simulink model "CAR_CONTROL_SYSTEM"  (R2024b)
settings: Solver=FixedStepAuto  StartTime=0.0  StopTime=inf  FixedStep=1e-3  RelTol=1e-3  EnableMultiTasking=on
model workspace (MAT data in the model file):
  SL_ROS_VariableLengthArrays_MaxSizes : object (value not decoded)
undefined symbols (not defined in the file or in its folder): angular, CIRCUIT, CLTF_DAMP, CLTF_FREQ, CLTF_GAIN, CONTROL, CONTROL_INI, DiscIntNeverNeededParam, dspblkCoreblockFVToolHelper, gcbh, INPUT, linear, MCP3201, MD25, MODEL, MODEL_INI, mpcstate, MPU60X0, MPU9250, MSG, NAV_MPC_CONTROL, OUTPUT, SAMPLING_TIME, SYSID_INPUT, VL6180X
libraries: raspberrypiCommlib x153, simulink x85, raspberrypiNetworklib x8, embedlinuxBasiclib x6, ctrlSharedLib x2, ros2lib x2, mpclib x1, vrlib x1, sldrtlib x1
(part 8 of 16)

== system CAR_CONTROL_SYSTEM/HARDWARE/SENSORS/WALL RANGE SENSOR/VL6180X_I2C_FRONT/VL6180X INITIALIZATION/MEASUREMENT CONFIGURATION/START READ RANGE CONTINUOUS ==
  Enable : EnablePort
  Constant2 : Constant  Value=hex2dec('03')  OutDataTypeStr=uint8  SampleTime=SAMPLING_TIME
  I2C WRITE: SYSRANGE_START : Subsystem  mask{SLAVE_ADDRESS=VL6180X.ADDRESS, REGISTER_ADDRESS=VL6180X.SYSRANGE_START}
      mask prompts: SLAVE_ADDRESS "SLAVE ADDRESS"; REGISTER_ADDRESS "REGISTER ADDRESS"
      mask init:
      | REGISTER_ADDRESS_MSB = uint8(floor(REGISTER_ADDRESS/(2^8)));
      | REGISTER_ADDRESS_LSB = uint8(rem(REGISTER_ADDRESS,2^8));
  wires:
  Constant2/1 -> I2C WRITE: SYSRANGE_START/1(DATA)

== system CAR_CONTROL_SYSTEM/HARDWARE/SENSORS/WALL RANGE SENSOR/VL6180X_I2C_FRONT/VL6180X INITIALIZATION/MEASUREMENT CONFIGURATION/START READ RANGE SINGLE ==
  Enable : EnablePort
  Constant1 : Constant  Value=hex2dec('01')  OutDataTypeStr=uint8  SampleTime=SAMPLING_TIME
  I2C WRITE: SYSRANGE_START : Subsystem  mask{SLAVE_ADDRESS=VL6180X.ADDRESS, REGISTER_ADDRESS=VL6180X.SYSRANGE_START}
      mask prompts: SLAVE_ADDRESS "SLAVE ADDRESS"; REGISTER_ADDRESS "REGISTER ADDRESS"
      mask init:
      | REGISTER_ADDRESS_MSB = uint8(floor(REGISTER_ADDRESS/(2^8)));
      | REGISTER_ADDRESS_LSB = uint8(rem(REGISTER_ADDRESS,2^8));
  wires:
  Constant1/1 -> I2C WRITE: SYSRANGE_START/1(DATA)

== system CAR_CONTROL_SYSTEM/HARDWARE/SENSORS/WALL RANGE SENSOR/VL6180X_I2C_FRONT/VL6180X INITIALIZATION/OTHER SPECIFIC SETTINGS (OPTIONAL)/I2C WRITE: INTERLEAVED_MODE_ENABLE ==
  DATA : Inport
  Constant : Constant  Value=REGISTER_ADDRESS_MSB  OutDataTypeStr=uint8  SampleTime=SAMPLING_TIME
  Constant1 : Constant  Value=REGISTER_ADDRESS_LSB  OutDataTypeStr=uint8  SampleTime=SAMPLING_TIME
  Mux : Mux  Inputs=3
  REGISTER ADDRESS : raspberrypiCommlib/I2C Controller Write  Priority=10  BoardProperty=Pi 3 Model B+  I2CModule=1  Mode=Master  SlaveAddress=SLAVE_ADDRESS  SlaveByteOrder=BigEndian  Direction=Transmitter  RegisterAddressMode=off  RegisterAddress=hex2dec('207')  SlaveDataType=uint8  DataLength=1  NoAck=off  RepeatedStart=off  OutputStatus=off
  wires:
  Mux/1 -> REGISTER ADDRESS/1
  Constant/1 -> Mux/1
  DATA/1 -> Mux/3
  Constant1/1 -> Mux/2

== system CAR_CONTROL_SYSTEM/HARDWARE/SENSORS/WALL RANGE SENSOR/VL6180X_I2C_FRONT/VL6180X INITIALIZATION/OTHER SPECIFIC SETTINGS (OPTIONAL)/I2C WRITE: SYSRANGE_MAX_CONVERGENCE_TIME ==
  DATA : Inport
  Constant : Constant  Value=REGISTER_ADDRESS_MSB  OutDataTypeStr=uint8  SampleTime=SAMPLING_TIME
  Constant1 : Constant  Value=REGISTER_ADDRESS_LSB  OutDataTypeStr=uint8  SampleTime=SAMPLING_TIME
  Mux : Mux  Inputs=3
  REGISTER ADDRESS : raspberrypiCommlib/I2C Controller Write  Priority=10  BoardProperty=Pi 3 Model B+  I2CModule=1  Mode=Master  SlaveAddress=SLAVE_ADDRESS  SlaveByteOrder=BigEndian  Direction=Transmitter  RegisterAddressMode=off  RegisterAddress=hex2dec('207')  SlaveDataType=uint8  DataLength=1  NoAck=off  RepeatedStart=off  OutputStatus=off
  wires:
  Mux/1 -> REGISTER ADDRESS/1
  Constant/1 -> Mux/1
  DATA/1 -> Mux/3
  Constant1/1 -> Mux/2

== system CAR_CONTROL_SYSTEM/HARDWARE/SENSORS/WALL RANGE SENSOR/VL6180X_I2C_REAR/READ RANGE/CHECK READOUT/SENSOR INITIALIZATION ==
  Enable : EnablePort
  Data Store Write1 : DataStoreWrite  DataStoreName=VL6180X_COUNTER  IndexOptions=Index vector (dialog)  Indices=1  OutputSizes=1
  Data Store Write2 : DataStoreWrite  Priority=100  DataStoreName=VL6180X_STATUS  IndexOptions=Index vector (dialog)  Indices=1  OutputSizes=1
  INITIALIZATION : Constant  Value=0  OutDataTypeStr=uint8  SampleTime=SAMPLING_TIME
  READY1 : Constant  Value=0  OutDataTypeStr=uint8  SampleTime=SAMPLING_TIME
  wires:
  INITIALIZATION/1 -> Data Store Write2/1
  READY1/1 -> Data Store Write1/1

== system CAR_CONTROL_SYSTEM/HARDWARE/SENSORS/WALL RANGE SENSOR/VL6180X_I2C_REAR/READ RANGE/READ RANGE VALUE/I2C READ: VL6180X.RESULT_RANGE_VAL ==
  Constant : Constant  Value=REGISTER_ADDRESS  OutDataTypeStr=uint16  SampleTime=SAMPLING_TIME
  DATA TO BE READ : raspberrypiCommlib/I2C Controller Read  Priority=20  BoardProperty=Pi 3 Model B  I2CModule=1  Mode=Master  SlaveAddress=SLAVE_ADDRESS  SlaveByteOrder=BigEndian  Direction=Receiver  RegisterAddressMode=off  RegisterAddress=0  SlaveDataType=uint8  DataLength=uint8(N)  NoAck=off  RepeatedStart=off  OutputStatus=off  SampleTime=SAMPLING_TIME
  REGISTER ADDRESS : raspberrypiCommlib/I2C Controller Write  Priority=10  BoardProperty=Pi 3 Model B  I2CModule=1  Mode=Master  SlaveAddress=SLAVE_ADDRESS  SlaveByteOrder=BigEndian  Direction=Transmitter  RegisterAddressMode=off  RegisterAddress=hex2dec('207')  SlaveDataType=uint8  DataLength=1  NoAck=off  RepeatedStart=off  OutputStatus=off
  DATA : Outport  VectorParamsAs1DForOutWhenUnconnected=off
  wires:
  DATA TO BE READ/1 -> DATA/1
  Constant/1 -> REGISTER ADDRESS/1

== system CAR_CONTROL_SYSTEM/HARDWARE/SENSORS/WALL RANGE SENSOR/VL6180X_I2C_REAR/READ RANGE/READ RANGE VALUE/I2C WRITE: SYSTEM_INTERRUPT_CLEAR ==
  DATA : Inport
  Constant : Constant  Value=REGISTER_ADDRESS_MSB  OutDataTypeStr=uint8  SampleTime=SAMPLING_TIME
  Constant1 : Constant  Value=REGISTER_ADDRESS_LSB  OutDataTypeStr=uint8  SampleTime=SAMPLING_TIME
  Mux : Mux  Inputs=3
  REGISTER ADDRESS : raspberrypiCommlib/I2C Controller Write  Priority=10  BoardProperty=Pi 3 Model B  I2CModule=1  Mode=Master  SlaveAddress=SLAVE_ADDRESS  SlaveByteOrder=BigEndian  Direction=Transmitter  RegisterAddressMode=off  RegisterAddress=hex2dec('207')  SlaveDataType=uint8  DataLength=1  NoAck=off  RepeatedStart=off  OutputStatus=off
  wires:
  Constant1/1 -> Mux/2
  DATA/1 -> Mux/3
  Constant/1 -> Mux/1
  Mux/1 -> REGISTER ADDRESS/1

== system CAR_CONTROL_SYSTEM/HARDWARE/SENSORS/WALL RANGE SENSOR/VL6180X_I2C_REAR/READ RANGE/START READ RANGE SINGLE/I2C WRITE: SYSRANGE_START ==
  DATA : Inport
  Constant : Constant  Value=REGISTER_ADDRESS_MSB  OutDataTypeStr=uint8  SampleTime=SAMPLING_TIME
  Constant1 : Constant  Value=REGISTER_ADDRESS_LSB  OutDataTypeStr=uint8  SampleTime=SAMPLING_TIME
  Mux : Mux  Inputs=3
  REGISTER ADDRESS : raspberrypiCommlib/I2C Controller Write  Priority=10  BoardProperty=Pi 3 Model B  I2CModule=1  Mode=Master  SlaveAddress=SLAVE_ADDRESS  SlaveByteOrder=BigEndian  Direction=Transmitter  RegisterAddressMode=off  RegisterAddress=hex2dec('207')  SlaveDataType=uint8  DataLength=1  NoAck=off  RepeatedStart=off  OutputStatus=off
  wires:
  Constant1/1 -> Mux/2
  DATA/1 -> Mux/3
  Constant/1 -> Mux/1
  Mux/1 -> REGISTER ADDRESS/1

== system CAR_CONTROL_SYSTEM/HARDWARE/SENSORS/WALL RANGE SENSOR/VL6180X_I2C_REAR/VL6180X INITIALIZATION/CHECK INITIALIZATION/I2C READ: SYSALS_INTEGRATION_PERIOD ==
  Constant : Constant  Value=REGISTER_ADDRESS  OutDataTypeStr=uint16  SampleTime=SAMPLING_TIME
  DATA TO BE READ : raspberrypiCommlib/I2C Controller Read  Priority=20  BoardProperty=Pi 3 Model B+  I2CModule=1  Mode=Master  SlaveAddress=SLAVE_ADDRESS  SlaveByteOrder=BigEndian  Direction=Receiver  RegisterAddressMode=off  RegisterAddress=0  SlaveDataType=uint8  DataLength=uint8(N)  NoAck=off  RepeatedStart=off  OutputStatus=off  SampleTime=SAMPLING_TIME
  REGISTER ADDRESS : raspberrypiCommlib/I2C Controller Write  Priority=10  BoardProperty=Pi 3 Model B+  I2CModule=1  Mode=Master  SlaveAddress=SLAVE_ADDRESS  SlaveByteOrder=BigEndian  Direction=Transmitter  RegisterAddressMode=off  RegisterAddress=hex2dec('207')  SlaveDataType=uint8  DataLength=1  NoAck=off  RepeatedStart=off  OutputStatus=off
  DATA : Outport  VectorParamsAs1DForOutWhenUnconnected=off
  wires:
  DATA TO BE READ/1 -> DATA/1
  Constant/1 -> REGISTER ADDRESS/1

== system CAR_CONTROL_SYSTEM/HARDWARE/SENSORS/WALL RANGE SENSOR/VL6180X_I2C_REAR/VL6180X INITIALIZATION/CHECK INITIALIZATION/I2C READ: SYSRANGE_MAX_CONVERGENCE_TIME ==
  Constant : Constant  Value=REGISTER_ADDRESS  OutDataTypeStr=uint16  SampleTime=SAMPLING_TIME
  DATA TO BE READ : raspberrypiCommlib/I2C Controller Read  Priority=20  BoardProperty=Pi 3 Model B  I2CModule=1  Mode=Master  SlaveAddress=SLAVE_ADDRESS  SlaveByteOrder=BigEndian  Direction=Receiver  RegisterAddressMode=off  RegisterAddress=0  SlaveDataType=uint8  DataLength=uint8(N)  NoAck=off  RepeatedStart=off  OutputStatus=off  SampleTime=SAMPLING_TIME
  REGISTER ADDRESS : raspberrypiCommlib/I2C Controller Write  Priority=10  BoardProperty=Pi 3 Model B  I2CModule=1  Mode=Master  SlaveAddress=SLAVE_ADDRESS  SlaveByteOrder=BigEndian  Direction=Transmitter  RegisterAddressMode=off  RegisterAddress=hex2dec('207')  SlaveDataType=uint8  DataLength=1  NoAck=off  RepeatedStart=off  OutputStatus=off
  DATA : Outport  VectorParamsAs1DForOutWhenUnconnected=off
  wires:
  Constant/1 -> REGISTER ADDRESS/1
  DATA TO BE READ/1 -> DATA/1

== system CAR_CONTROL_SYSTEM/HARDWARE/SENSORS/WALL RANGE SENSOR/VL6180X_I2C_REAR/VL6180X INITIALIZATION/CHECK INITIALIZATION/I2C READ: 0x1A7  ==
  Constant : Constant  Value=REGISTER_ADDRESS  OutDataTypeStr=uint16  SampleTime=SAMPLING_TIME
  DATA TO BE READ : raspberrypiCommlib/I2C Controller Read  Priority=20  BoardProperty=Pi 3 Model B+  I2CModule=1  Mode=Master  SlaveAddress=SLAVE_ADDRESS  SlaveByteOrder=BigEndian  Direction=Receiver  RegisterAddressMode=off  RegisterAddress=0  SlaveDataType=uint8  DataLength=uint8(N)  NoAck=off  RepeatedStart=off  OutputStatus=off  SampleTime=SAMPLING_TIME
  REGISTER ADDRESS : raspberrypiCommlib/I2C Controller Write  Priority=10  BoardProperty=Pi 3 Model B+  I2CModule=1  Mode=Master  SlaveAddress=SLAVE_ADDRESS  SlaveByteOrder=BigEndian  Direction=Transmitter  RegisterAddressMode=off  RegisterAddress=hex2dec('207')  SlaveDataType=uint8  DataLength=1  NoAck=off  RepeatedStart=off  OutputStatus=off
  DATA : Outport  VectorParamsAs1DForOutWhenUnconnected=off
  wires:
  DATA TO BE READ/1 -> DATA/1
  Constant/1 -> REGISTER ADDRESS/1

== system CAR_CONTROL_SYSTEM/HARDWARE/SENSORS/WALL RANGE SENSOR/VL6180X_I2C_REAR/VL6180X INITIALIZATION/CHECK INITIALIZATION/I2C WRITE: SYSTEM_INTERRUPT_CONFIG_GPIO ==
  Constant : Constant  Value=REGISTER_ADDRESS  OutDataTypeStr=uint16  SampleTime=SAMPLING_TIME
  DATA TO BE READ : raspberrypiCommlib/I2C Controller Read  Priority=20  BoardProperty=Pi 3 Model B+  I2CModule=1  Mode=Master  SlaveAddress=SLAVE_ADDRESS  SlaveByteOrder=BigEndian  Direction=Receiver  RegisterAddressMode=off  RegisterAddress=0  SlaveDataType=uint8  DataLength=uint8(N)  NoAck=off  RepeatedStart=off  OutputStatus=off  SampleTime=SAMPLING_TIME
  REGISTER ADDRESS : raspberrypiCommlib/I2C Controller Write  Priority=10  BoardProperty=Pi 3 Model B+  I2CModule=1  Mode=Master  SlaveAddress=SLAVE_ADDRESS  SlaveByteOrder=BigEndian  Direction=Transmitter  RegisterAddressMode=off  RegisterAddress=hex2dec('207')  SlaveDataType=uint8  DataLength=1  NoAck=off  RepeatedStart=off  OutputStatus=off
  DATA : Outport  VectorParamsAs1DForOutWhenUnconnected=off
  wires:
  DATA TO BE READ/1 -> DATA/1
  Constant/1 -> REGISTER ADDRESS/1

== system CAR_CONTROL_SYSTEM/HARDWARE/SENSORS/WALL RANGE SENSOR/VL6180X_I2C_REAR/VL6180X INITIALIZATION/LOAD PRIVATE REGISTERS (MANDATORY)/I2C WRITE: 0x030  ==
  DATA : Inport
  Constant : Constant  Value=REGISTER_ADDRESS_MSB  OutDataTypeStr=uint8  SampleTime=SAMPLING_TIME
  Constant1 : Constant  Value=REGISTER_ADDRESS_LSB  OutDataTypeStr=uint8  SampleTime=SAMPLING_TIME
  Mux : Mux  Inputs=3
  REGISTER ADDRESS : raspberrypiCommlib/I2C Controller Write  Priority=10  BoardProperty=Pi 3 Model B+  I2CModule=1  Mode=Master  SlaveAddress=SLAVE_ADDRESS  SlaveByteOrder=BigEndian  Direction=Transmitter  RegisterAddressMode=off  RegisterAddress=hex2dec('207')  SlaveDataType=uint8  DataLength=1  NoAck=off  RepeatedStart=off  OutputStatus=off
  wires:
  Constant1/1 -> Mux/2
  DATA/1 -> Mux/3
  Constant/1 -> Mux/1
  Mux/1 -> REGISTER ADDRESS/1

== system CAR_CONTROL_SYSTEM/HARDWARE/SENSORS/WALL RANGE SENSOR/VL6180X_I2C_REAR/VL6180X INITIALIZATION/LOAD PRIVATE REGISTERS (MANDATORY)/I2C WRITE: 0x096 ==
  DATA : Inport
  Constant : Constant  Value=REGISTER_ADDRESS_MSB  OutDataTypeStr=uint8  SampleTime=SAMPLING_TIME
  Constant1 : Constant  Value=REGISTER_ADDRESS_LSB  OutDataTypeStr=uint8  SampleTime=SAMPLING_TIME
  Mux : Mux  Inputs=3
  REGISTER ADDRESS : raspberrypiCommlib/I2C Controller Write  Priority=10  BoardProperty=Pi 3 Model B+  I2CModule=1  Mode=Master  SlaveAddress=SLAVE_ADDRESS  SlaveByteOrder=BigEndian  Direction=Transmitter  RegisterAddressMode=off  RegisterAddress=hex2dec('207')  SlaveDataType=uint8  DataLength=1  NoAck=off  RepeatedStart=off  OutputStatus=off
  wires:
  Constant1/1 -> Mux/2
  DATA/1 -> Mux/3
  Constant/1 -> Mux/1
  Mux/1 -> REGISTER ADDRESS/1

== system CAR_CONTROL_SYSTEM/HARDWARE/SENSORS/WALL RANGE SENSOR/VL6180X_I2C_REAR/VL6180X INITIALIZATION/LOAD PRIVATE REGISTERS (MANDATORY)/I2C WRITE: 0x097 ==
  DATA : Inport
  Constant : Constant  Value=REGISTER_ADDRESS_MSB  OutDataTypeStr=uint8  SampleTime=SAMPLING_TIME
  Constant1 : Constant  Value=REGISTER_ADDRESS_LSB  OutDataTypeStr=uint8  SampleTime=SAMPLING_TIME
  Mux : Mux  Inputs=3
  REGISTER ADDRESS : raspberrypiCommlib/I2C Controller Write  Priority=10  BoardProperty=Pi 3 Model B+  I2CModule=1  Mode=Master  SlaveAddress=SLAVE_ADDRESS  SlaveByteOrder=BigEndian  Direction=Transmitter  RegisterAddressMode=off  RegisterAddress=hex2dec('207')  SlaveDataType=uint8  DataLength=1  NoAck=off  RepeatedStart=off  OutputStatus=off
  wires:
  Constant1/1 -> Mux/2
  DATA/1 -> Mux/3
  Constant/1 -> Mux/1
  Mux/1 -> REGISTER ADDRESS/1

== system CAR_CONTROL_SYSTEM/HARDWARE/SENSORS/WALL RANGE SENSOR/VL6180X_I2C_REAR/VL6180X INITIALIZATION/LOAD PRIVATE REGISTERS (MANDATORY)/I2C WRITE: 0x09F ==
  DATA : Inport
  Constant : Constant  Value=REGISTER_ADDRESS_MSB  OutDataTypeStr=uint8  SampleTime=SAMPLING_TIME
  Constant1 : Constant  Value=REGISTER_ADDRESS_LSB  OutDataTypeStr=uint8  SampleTime=SAMPLING_TIME
  Mux : Mux  Inputs=3
  REGISTER ADDRESS : raspberrypiCommlib/I2C Controller Write  Priority=10  BoardProperty=Pi 3 Model B+  I2CModule=1  Mode=Master  SlaveAddress=SLAVE_ADDRESS  SlaveByteOrder=BigEndian  Direction=Transmitter  RegisterAddressMode=off  RegisterAddress=hex2dec('207')  SlaveDataType=uint8  DataLength=1  NoAck=off  RepeatedStart=off  OutputStatus=off
  wires:
  Constant1/1 -> Mux/2
  DATA/1 -> Mux/3
  Constant/1 -> Mux/1
  Mux/1 -> REGISTER ADDRESS/1

== system CAR_CONTROL_SYSTEM/HARDWARE/SENSORS/WALL RANGE SENSOR/VL6180X_I2C_REAR/VL6180X INITIALIZATION/LOAD PRIVATE REGISTERS (MANDATORY)/I2C WRITE: 0x0A3 ==
  DATA : Inport
  Constant : Constant  Value=REGISTER_ADDRESS_MSB  OutDataTypeStr=uint8  SampleTime=SAMPLING_TIME
  Constant1 : Constant  Value=REGISTER_ADDRESS_LSB  OutDataTypeStr=uint8  SampleTime=SAMPLING_TIME
  Mux : Mux  Inputs=3
  REGISTER ADDRESS : raspberrypiCommlib/I2C Controller Write  Priority=10  BoardProperty=Pi 3 Model B+  I2CModule=1  Mode=Master  SlaveAddress=SLAVE_ADDRESS  SlaveByteOrder=BigEndian  Direction=Transmitter  RegisterAddressMode=off  RegisterAddress=hex2dec('207')  SlaveDataType=uint8  DataLength=1  NoAck=off  RepeatedStart=off  OutputStatus=off
  wires:
  Constant1/1 -> Mux/2
  DATA/1 -> Mux/3
  Constant/1 -> Mux/1
  Mux/1 -> REGISTER ADDRESS/1

== system CAR_CONTROL_SYSTEM/HARDWARE/SENSORS/WALL RANGE SENSOR/VL6180X_I2C_REAR/VL6180X INITIALIZATION/LOAD PRIVATE REGISTERS (MANDATORY)/I2C WRITE: 0x0B2 ==
  DATA : Inport
  Constant : Constant  Value=REGISTER_ADDRESS_MSB  OutDataTypeStr=uint8  SampleTime=SAMPLING_TIME
  Constant1 : Constant  Value=REGISTER_ADDRESS_LSB  OutDataTypeStr=uint8  SampleTime=SAMPLING_TIME
  Mux : Mux  Inputs=3
  REGISTER ADDRESS : raspberrypiCommlib/I2C Controller Write  Priority=10  BoardProperty=Pi 3 Model B+  I2CModule=1  Mode=Master  SlaveAddress=SLAVE_ADDRESS  SlaveByteOrder=BigEndian  Direction=Transmitter  RegisterAddressMode=off  RegisterAddress=hex2dec('207')  SlaveDataType=uint8  DataLength=1  NoAck=off  RepeatedStart=off  OutputStatus=off
  wires:
  Constant1/1 -> Mux/2
  DATA/1 -> Mux/3
  Constant/1 -> Mux/1
  Mux/1 -> REGISTER ADDRESS/1

== system CAR_CONTROL_SYSTEM/HARDWARE/SENSORS/WALL RANGE SENSOR/VL6180X_I2C_REAR/VL6180X INITIALIZATION/LOAD PRIVATE REGISTERS (MANDATORY)/I2C WRITE: 0x0B7 ==
  DATA : Inport
  Constant : Constant  Value=REGISTER_ADDRESS_MSB  OutDataTypeStr=uint8  SampleTime=SAMPLING_TIME
  Constant1 : Constant  Value=REGISTER_ADDRESS_LSB  OutDataTypeStr=uint8  SampleTime=SAMPLING_TIME
  Mux : Mux  Inputs=3
  REGISTER ADDRESS : raspberrypiCommlib/I2C Controller Write  Priority=10  BoardProperty=Pi 3 Model B+  I2CModule=1  Mode=Master  SlaveAddress=SLAVE_ADDRESS  SlaveByteOrder=BigEndian  Direction=Transmitter  RegisterAddressMode=off  RegisterAddress=hex2dec('207')  SlaveDataType=uint8  DataLength=1  NoAck=off  RepeatedStart=off  OutputStatus=off
  wires:
  Constant1/1 -> Mux/2
  DATA/1 -> Mux/3
  Constant/1 -> Mux/1
  Mux/1 -> REGISTER ADDRESS/1

== system CAR_CONTROL_SYSTEM/HARDWARE/SENSORS/WALL RANGE SENSOR/VL6180X_I2C_REAR/VL6180X INITIALIZATION/LOAD PRIVATE REGISTERS (MANDATORY)/I2C WRITE: 0x0BB ==
  DATA : Inport
  Constant : Constant  Value=REGISTER_ADDRESS_MSB  OutDataTypeStr=uint8  SampleTime=SAMPLING_TIME
  Constant1 : Constant  Value=REGISTER_ADDRESS_LSB  OutDataTypeStr=uint8  SampleTime=SAMPLING_TIME
  Mux : Mux  Inputs=3
  REGISTER ADDRESS : raspberrypiCommlib/I2C Controller Write  Priority=10  BoardProperty=Pi 3 Model B+  I2CModule=1  Mode=Master  SlaveAddress=SLAVE_ADDRESS  SlaveByteOrder=BigEndian  Direction=Transmitter  RegisterAddressMode=off  RegisterAddress=hex2dec('207')  SlaveDataType=uint8  DataLength=1  NoAck=off  RepeatedStart=off  OutputStatus=off
  wires:
  Constant1/1 -> Mux/2
  DATA/1 -> Mux/3
  Constant/1 -> Mux/1
  Mux/1 -> REGISTER ADDRESS/1

== system CAR_CONTROL_SYSTEM/HARDWARE/SENSORS/WALL RANGE SENSOR/VL6180X_I2C_REAR/VL6180X INITIALIZATION/LOAD PRIVATE REGISTERS (MANDATORY)/I2C WRITE: 0x0CA ==
  DATA : Inport
  Constant : Constant  Value=REGISTER_ADDRESS_MSB  OutDataTypeStr=uint8  SampleTime=SAMPLING_TIME
  Constant1 : Constant  Value=REGISTER_ADDRESS_LSB  OutDataTypeStr=uint8  SampleTime=SAMPLING_TIME
  Mux : Mux  Inputs=3
  REGISTER ADDRESS : raspberrypiCommlib/I2C Controller Write  Priority=10  BoardProperty=Pi 3 Model B+  I2CModule=1  Mode=Master  SlaveAddress=SLAVE_ADDRESS  SlaveByteOrder=BigEndian  Direction=Transmitter  RegisterAddressMode=off  RegisterAddress=hex2dec('207')  SlaveDataType=uint8  DataLength=1  NoAck=off  RepeatedStart=off  OutputStatus=off
  wires:
  Constant1/1 -> Mux/2
  DATA/1 -> Mux/3
  Constant/1 -> Mux/1
  Mux/1 -> REGISTER ADDRESS/1

== system CAR_CONTROL_SYSTEM/HARDWARE/SENSORS/WALL RANGE SENSOR/VL6180X_I2C_REAR/VL6180X INITIALIZATION/LOAD PRIVATE REGISTERS (MANDATORY)/I2C WRITE: 0x0D9 ==
  DATA : Inport
  Constant : Constant  Value=REGISTER_ADDRESS_MSB  OutDataTypeStr=uint8  SampleTime=SAMPLING_TIME
  Constant1 : Constant  Value=REGISTER_ADDRESS_LSB  OutDataTypeStr=uint8  SampleTime=SAMPLING_TIME
  Mux : Mux  Inputs=3
  REGISTER ADDRESS : raspberrypiCommlib/I2C Controller Write  Priority=10  BoardProperty=Pi 3 Model B+  I2CModule=1  Mode=Master  SlaveAddress=SLAVE_ADDRESS  SlaveByteOrder=BigEndian  Direction=Transmitter  RegisterAddressMode=off  RegisterAddress=hex2dec('207')  SlaveDataType=uint8  DataLength=1  NoAck=off  RepeatedStart=off  OutputStatus=off
  wires:
  Constant1/1 -> Mux/2
  DATA/1 -> Mux/3
  Constant/1 -> Mux/1
  Mux/1 -> REGISTER ADDRESS/1

== system CAR_CONTROL_SYSTEM/HARDWARE/SENSORS/WALL RANGE SENSOR/VL6180X_I2C_REAR/VL6180X INITIALIZATION/LOAD PRIVATE REGISTERS (MANDATORY)/I2C WRITE: 0x0DB ==
  DATA : Inport
  Constant : Constant  Value=REGISTER_ADDRESS_MSB  OutDataTypeStr=uint8  SampleTime=SAMPLING_TIME
  Constant1 : Constant  Value=REGISTER_ADDRESS_LSB  OutDataTypeStr=uint8  SampleTime=SAMPLING_TIME
  Mux : Mux  Inputs=3
  REGISTER ADDRESS : raspberrypiCommlib/I2C Controller Write  Priority=10  BoardProperty=Pi 3 Model B+  I2CModule=1  Mode=Master  SlaveAddress=SLAVE_ADDRESS  SlaveByteOrder=BigEndian  Direction=Transmitter  RegisterAddressMode=off  RegisterAddress=hex2dec('207')  SlaveDataType=uint8  DataLength=1  NoAck=off  RepeatedStart=off  OutputStatus=off
  wires:
  Constant1/1 -> Mux/2
  DATA/1 -> Mux/3
  Constant/1 -> Mux/1
  Mux/1 -> REGISTER ADDRESS/1

== system CAR_CONTROL_SYSTEM/HARDWARE/SENSORS/WALL RANGE SENSOR/VL6180X_I2C_REAR/VL6180X INITIALIZATION/LOAD PRIVATE REGISTERS (MANDATORY)/I2C WRITE: 0x0DC ==
  DATA : Inport
  Constant : Constant  Value=REGISTER_ADDRESS_MSB  OutDataTypeStr=uint8  SampleTime=SAMPLING_TIME
  Constant1 : Constant  Value=REGISTER_ADDRESS_LSB  OutDataTypeStr=uint8  SampleTime=SAMPLING_TIME
  Mux : Mux  Inputs=3
  REGISTER ADDRESS : raspberrypiCommlib/I2C Controller Write  Priority=10  BoardProperty=Pi 3 Model B+  I2CModule=1  Mode=Master  SlaveAddress=SLAVE_ADDRESS  SlaveByteOrder=BigEndian  Direction=Transmitter  RegisterAddressMode=off  RegisterAddress=hex2dec('207')  SlaveDataType=uint8  DataLength=1  NoAck=off  RepeatedStart=off  OutputStatus=off
  wires:
  Constant1/1 -> Mux/2
  DATA/1 -> Mux/3
  Constant/1 -> Mux/1
  Mux/1 -> REGISTER ADDRESS/1

== system CAR_CONTROL_SYSTEM/HARDWARE/SENSORS/WALL RANGE SENSOR/VL6180X_I2C_REAR/VL6180X INITIALIZATION/LOAD PRIVATE REGISTERS (MANDATORY)/I2C WRITE: 0x0DD ==
  DATA : Inport
  Constant : Constant  Value=REGISTER_ADDRESS_MSB  OutDataTypeStr=uint8  SampleTime=SAMPLING_TIME
  Constant1 : Constant  Value=REGISTER_ADDRESS_LSB  OutDataTypeStr=uint8  SampleTime=SAMPLING_TIME
  Mux : Mux  Inputs=3
  REGISTER ADDRESS : raspberrypiCommlib/I2C Controller Write  Priority=10  BoardProperty=Pi 3 Model B+  I2CModule=1  Mode=Master  SlaveAddress=SLAVE_ADDRESS  SlaveByteOrder=BigEndian  Direction=Transmitter  RegisterAddressMode=off  RegisterAddress=hex2dec('207')  SlaveDataType=uint8  DataLength=1  NoAck=off  RepeatedStart=off  OutputStatus=off
  wires:
  Constant1/1 -> Mux/2
  DATA/1 -> Mux/3
  Constant/1 -> Mux/1
  Mux/1 -> REGISTER ADDRESS/1

== system CAR_CONTROL_SYSTEM/HARDWARE/SENSORS/WALL RANGE SENSOR/VL6180X_I2C_REAR/VL6180X INITIALIZATION/LOAD PRIVATE REGISTERS (MANDATORY)/I2C WRITE: 0x0E3 ==
  DATA : Inport
  Constant : Constant  Value=REGISTER_ADDRESS_MSB  OutDataTypeStr=uint8  SampleTime=SAMPLING_TIME
  Constant1 : Constant  Value=REGISTER_ADDRESS_LSB  OutDataTypeStr=uint8  SampleTime=SAMPLING_TIME
  Mux : Mux  Inputs=3
  REGISTER ADDRESS : raspberrypiCommlib/I2C Controller Write  Priority=10  BoardProperty=Pi 3 Model B+  I2CModule=1  Mode=Master  SlaveAddress=SLAVE_ADDRESS  SlaveByteOrder=BigEndian  Direction=Transmitter  RegisterAddressMode=off  RegisterAddress=hex2dec('207')  SlaveDataType=uint8  DataLength=1  NoAck=off  RepeatedStart=off  OutputStatus=off
  wires:
  Constant1/1 -> Mux/2
  DATA/1 -> Mux/3
  Constant/1 -> Mux/1
  Mux/1 -> REGISTER ADDRESS/1

== system CAR_CONTROL_SYSTEM/HARDWARE/SENSORS/WALL RANGE SENSOR/VL6180X_I2C_REAR/VL6180X INITIALIZATION/LOAD PRIVATE REGISTERS (MANDATORY)/I2C WRITE: 0x0E4 ==
  DATA : Inport
  Constant : Constant  Value=REGISTER_ADDRESS_MSB  OutDataTypeStr=uint8  SampleTime=SAMPLING_TIME
  Constant1 : Constant  Value=REGISTER_ADDRESS_LSB  OutDataTypeStr=uint8  SampleTime=SAMPLING_TIME
  Mux : Mux  Inputs=3
  REGISTER ADDRESS : raspberrypiCommlib/I2C Controller Write  Priority=10  BoardProperty=Pi 3 Model B+  I2CModule=1  Mode=Master  SlaveAddress=SLAVE_ADDRESS  SlaveByteOrder=BigEndian  Direction=Transmitter  RegisterAddressMode=off  RegisterAddress=hex2dec('207')  SlaveDataType=uint8  DataLength=1  NoAck=off  RepeatedStart=off  OutputStatus=off
  wires:
  Constant1/1 -> Mux/2
  DATA/1 -> Mux/3
  Constant/1 -> Mux/1
  Mux/1 -> REGISTER ADDRESS/1

== system CAR_CONTROL_SYSTEM/HARDWARE/SENSORS/WALL RANGE SENSOR/VL6180X_I2C_REAR/VL6180X INITIALIZATION/LOAD PRIVATE REGISTERS (MANDATORY)/I2C WRITE: 0x0E5 ==
  DATA : Inport
  Constant : Constant  Value=REGISTER_ADDRESS_MSB  OutDataTypeStr=uint8  SampleTime=SAMPLING_TIME
  Constant1 : Constant  Value=REGISTER_ADDRESS_LSB  OutDataTypeStr=uint8  SampleTime=SAMPLING_TIME
  Mux : Mux  Inputs=3
  REGISTER ADDRESS : raspberrypiCommlib/I2C Controller Write  Priority=10  BoardProperty=Pi 3 Model B+  I2CModule=1  Mode=Master  SlaveAddress=SLAVE_ADDRESS  SlaveByteOrder=BigEndian  Direction=Transmitter  RegisterAddressMode=off  RegisterAddress=hex2dec('207')  SlaveDataType=uint8  DataLength=1  NoAck=off  RepeatedStart=off  OutputStatus=off
  wires:
  Constant1/1 -> Mux/2
  DATA/1 -> Mux/3
  Constant/1 -> Mux/1
  Mux/1 -> REGISTER ADDRESS/1

== system CAR_CONTROL_SYSTEM/HARDWARE/SENSORS/WALL RANGE SENSOR/VL6180X_I2C_REAR/VL6180X INITIALIZATION/LOAD PRIVATE REGISTERS (MANDATORY)/I2C WRITE: 0x0E6 ==
  DATA : Inport
  Constant : Constant  Value=REGISTER_ADDRESS_MSB  OutDataTypeStr=uint8  SampleTime=SAMPLING_TIME
  Constant1 : Constant  Value=REGISTER_ADDRESS_LSB  OutDataTypeStr=uint8  SampleTime=SAMPLING_TIME
  Mux : Mux  Inputs=3
  REGISTER ADDRESS : raspberrypiCommlib/I2C Controller Write  Priority=10  BoardProperty=Pi 3 Model B+  I2CModule=1  Mode=Master  SlaveAddress=SLAVE_ADDRESS  SlaveByteOrder=BigEndian  Direction=Transmitter  RegisterAddressMode=off  RegisterAddress=hex2dec('207')  SlaveDataType=uint8  DataLength=1  NoAck=off  RepeatedStart=off  OutputStatus=off
  wires:
  Constant1/1 -> Mux/2
  DATA/1 -> Mux/3
  Constant/1 -> Mux/1
  Mux/1 -> REGISTER ADDRESS/1

== system CAR_CONTROL_SYSTEM/HARDWARE/SENSORS/WALL RANGE SENSOR/VL6180X_I2C_REAR/VL6180X INITIALIZATION/LOAD PRIVATE REGISTERS (MANDATORY)/I2C WRITE: 0x0E7 ==
  DATA : Inport
  Constant : Constant  Value=REGISTER_ADDRESS_MSB  OutDataTypeStr=uint8  SampleTime=SAMPLING_TIME
  Constant1 : Constant  Value=REGISTER_ADDRESS_LSB  OutDataTypeStr=uint8  SampleTime=SAMPLING_TIME
  Mux : Mux  Inputs=3
  REGISTER ADDRESS : raspberrypiCommlib/I2C Controller Write  Priority=10  BoardProperty=Pi 3 Model B+  I2CModule=1  Mode=Master  SlaveAddress=SLAVE_ADDRESS  SlaveByteOrder=BigEndian  Direction=Transmitter  RegisterAddressMode=off  RegisterAddress=hex2dec('207')  SlaveDataType=uint8  DataLength=1  NoAck=off  RepeatedStart=off  OutputStatus=off
  wires:
  Constant1/1 -> Mux/2
  DATA/1 -> Mux/3
  Constant/1 -> Mux/1
  Mux/1 -> REGISTER ADDRESS/1

== system CAR_CONTROL_SYSTEM/HARDWARE/SENSORS/WALL RANGE SENSOR/VL6180X_I2C_REAR/VL6180X INITIALIZATION/LOAD PRIVATE REGISTERS (MANDATORY)/I2C WRITE: 0x0F5 ==
  DATA : Inport
  Constant : Constant  Value=REGISTER_ADDRESS_MSB  OutDataTypeStr=uint8  SampleTime=SAMPLING_TIME
  Constant1 : Constant  Value=REGISTER_ADDRESS_LSB  OutDataTypeStr=uint8  SampleTime=SAMPLING_TIME
  Mux : Mux  Inputs=3
  REGISTER ADDRESS : raspberrypiCommlib/I2C Controller Write  Priority=10  BoardProperty=Pi 3 Model B+  I2CModule=1  Mode=Master  SlaveAddress=SLAVE_ADDRESS  SlaveByteOrder=BigEndian  Direction=Transmitter  RegisterAddressMode=off  RegisterAddress=hex2dec('207')  SlaveDataType=uint8  DataLength=1  NoAck=off  RepeatedStart=off  OutputStatus=off
  wires:
  Constant1/1 -> Mux/2
  DATA/1 -> Mux/3
  Constant/1 -> Mux/1
  Mux/1 -> REGISTER ADDRESS/1

== system CAR_CONTROL_SYSTEM/HARDWARE/SENSORS/WALL RANGE SENSOR/VL6180X_I2C_REAR/VL6180X INITIALIZATION/LOAD PRIVATE REGISTERS (MANDATORY)/I2C WRITE: 0x0FF  ==
  DATA : Inport
  Constant : Constant  Value=REGISTER_ADDRESS_MSB  OutDataTypeStr=uint8  SampleTime=SAMPLING_TIME
  Constant1 : Constant  Value=REGISTER_ADDRESS_LSB  OutDataTypeStr=uint8  SampleTime=SAMPLING_TIME
  Mux : Mux  Inputs=3
  REGISTER ADDRESS : raspberrypiCommlib/I2C Controller Write  Priority=10  BoardProperty=Pi 3 Model B+  I2CModule=1  Mode=Master  SlaveAddress=SLAVE_ADDRESS  SlaveByteOrder=BigEndian  Direction=Transmitter  RegisterAddressMode=off  RegisterAddress=hex2dec('207')  SlaveDataType=uint8  DataLength=1  NoAck=off  RepeatedStart=off  OutputStatus=off
  wires:
  Constant1/1 -> Mux/2
  DATA/1 -> Mux/3
  Constant/1 -> Mux/1
  Mux/1 -> REGISTER ADDRESS/1

== system CAR_CONTROL_SYSTEM/HARDWARE/SENSORS/WALL RANGE SENSOR/VL6180X_I2C_REAR/VL6180X INITIALIZATION/LOAD PRIVATE REGISTERS (MANDATORY)/I2C WRITE: 0x100  ==
  DATA : Inport
  Constant : Constant  Value=REGISTER_ADDRESS_MSB  OutDataTypeStr=uint8  SampleTime=SAMPLING_TIME
  Constant1 : Constant  Value=REGISTER_ADDRESS_LSB  OutDataTypeStr=uint8  SampleTime=SAMPLING_TIME
  Mux : Mux  Inputs=3
  REGISTER ADDRESS : raspberrypiCommlib/I2C Controller Write  Priority=10  BoardProperty=Pi 3 Model B+  I2CModule=1  Mode=Master  SlaveAddress=SLAVE_ADDRESS  SlaveByteOrder=BigEndian  Direction=Transmitter  RegisterAddressMode=off  RegisterAddress=hex2dec('207')  SlaveDataType=uint8  DataLength=1  NoAck=off  RepeatedStart=off  OutputStatus=off
  wires:
  Constant1/1 -> Mux/2
  DATA/1 -> Mux/3
  Constant/1 -> Mux/1
  Mux/1 -> REGISTER ADDRESS/1

== system CAR_CONTROL_SYSTEM/HARDWARE/SENSORS/WALL RANGE SENSOR/VL6180X_I2C_REAR/VL6180X INITIALIZATION/LOAD PRIVATE REGISTERS (MANDATORY)/I2C WRITE: 0x198 ==
  DATA : Inport
  Constant : Constant  Value=REGISTER_ADDRESS_MSB  OutDataTypeStr=uint8  SampleTime=SAMPLING_TIME
  Constant1 : Constant  Value=REGISTER_ADDRESS_LSB  OutDataTypeStr=uint8  SampleTime=SAMPLING_TIME
  Mux : Mux  Inputs=3
  REGISTER ADDRESS : raspberrypiCommlib/I2C Controller Write  Priority=10  BoardProperty=Pi 3 Model B+  I2CModule=1  Mode=Master  SlaveAddress=SLAVE_ADDRESS  SlaveByteOrder=BigEndian  Direction=Transmitter  RegisterAddressMode=off  RegisterAddress=hex2dec('207')  SlaveDataType=uint8  DataLength=1  NoAck=off  RepeatedStart=off  OutputStatus=off
  wires:
  Constant1/1 -> Mux/2
  DATA/1 -> Mux/3
  Constant/1 -> Mux/1
  Mux/1 -> REGISTER ADDRESS/1

== system CAR_CONTROL_SYSTEM/HARDWARE/SENSORS/WALL RANGE SENSOR/VL6180X_I2C_REAR/VL6180X INITIALIZATION/LOAD PRIVATE REGISTERS (MANDATORY)/I2C WRITE: 0x199  ==
  DATA : Inport
  Constant : Constant  Value=REGISTER_ADDRESS_MSB  OutDataTypeStr=uint8  SampleTime=SAMPLING_TIME
  Constant1 : Constant  Value=REGISTER_ADDRESS_LSB  OutDataTypeStr=uint8  SampleTime=SAMPLING_TIME
  Mux : Mux  Inputs=3
  REGISTER ADDRESS : raspberrypiCommlib/I2C Controller Write  Priority=10  BoardProperty=Pi 3 Model B+  I2CModule=1  Mode=Master  SlaveAddress=SLAVE_ADDRESS  SlaveByteOrder=BigEndian  Direction=Transmitter  RegisterAddressMode=off  RegisterAddress=hex2dec('207')  SlaveDataType=uint8  DataLength=1  NoAck=off  RepeatedStart=off  OutputStatus=off
  wires:
  Constant1/1 -> Mux/2
  DATA/1 -> Mux/3
  Constant/1 -> Mux/1
  Mux/1 -> REGISTER ADDRESS/1

== system CAR_CONTROL_SYSTEM/HARDWARE/SENSORS/WALL RANGE SENSOR/VL6180X_I2C_REAR/VL6180X INITIALIZATION/LOAD PRIVATE REGISTERS (MANDATORY)/I2C WRITE: 0x1A6  ==
  DATA : Inport
  Constant : Constant  Value=REGISTER_ADDRESS_MSB  OutDataTypeStr=uint8  SampleTime=SAMPLING_TIME
  Constant1 : Constant  Value=REGISTER_ADDRESS_LSB  OutDataTypeStr=uint8  SampleTime=SAMPLING_TIME
  Mux : Mux  Inputs=3
  REGISTER ADDRESS : raspberrypiCommlib/I2C Controller Write  Priority=10  BoardProperty=Pi 3 Model B+  I2CModule=1  Mode=Master  SlaveAddress=SLAVE_ADDRESS  SlaveByteOrder=BigEndian  Direction=Transmitter  RegisterAddressMode=off  RegisterAddress=hex2dec('207')  SlaveDataType=uint8  DataLength=1  NoAck=off  RepeatedStart=off  OutputStatus=off
  wires:
  Constant1/1 -> Mux/2
  DATA/1 -> Mux/3
  Constant/1 -> Mux/1
  Mux/1 -> REGISTER ADDRESS/1

== system CAR_CONTROL_SYSTEM/HARDWARE/SENSORS/WALL RANGE SENSOR/VL6180X_I2C_REAR/VL6180X INITIALIZATION/LOAD PRIVATE REGISTERS (MANDATORY)/I2C WRITE: 0x1A7  ==
  DATA : Inport
  Constant : Constant  Value=REGISTER_ADDRESS_MSB  OutDataTypeStr=uint8  SampleTime=SAMPLING_TIME
  Constant1 : Constant  Value=REGISTER_ADDRESS_LSB  OutDataTypeStr=uint8  SampleTime=SAMPLING_TIME
  Mux : Mux  Inputs=3
  REGISTER ADDRESS : raspberrypiCommlib/I2C Controller Write  Priority=10  BoardProperty=Pi 3 Model B+  I2CModule=1  Mode=Master  SlaveAddress=SLAVE_ADDRESS  SlaveByteOrder=BigEndian  Direction=Transmitter  RegisterAddressMode=off  RegisterAddress=hex2dec('207')  SlaveDataType=uint8  DataLength=1  NoAck=off  RepeatedStart=off  OutputStatus=off
  wires:
  Constant1/1 -> Mux/2
  DATA/1 -> Mux/3
  Constant/1 -> Mux/1
  Mux/1 -> REGISTER ADDRESS/1

== system CAR_CONTROL_SYSTEM/HARDWARE/SENSORS/WALL RANGE SENSOR/VL6180X_I2C_REAR/VL6180X INITIALIZATION/LOAD PRIVATE REGISTERS (MANDATORY)/I2C WRITE: 0x1AC  ==
  DATA : Inport
  Constant : Constant  Value=REGISTER_ADDRESS_MSB  OutDataTypeStr=uint8  SampleTime=SAMPLING_TIME
  Constant1 : Constant  Value=REGISTER_ADDRESS_LSB  OutDataTypeStr=uint8  SampleTime=SAMPLING_TIME
  Mux : Mux  Inputs=3
  REGISTER ADDRESS : raspberrypiCommlib/I2C Controller Write  Priority=10  BoardProperty=Pi 3 Model B+  I2CModule=1  Mode=Master  SlaveAddress=SLAVE_ADDRESS  SlaveByteOrder=BigEndian  Direction=Transmitter  RegisterAddressMode=off  RegisterAddress=hex2dec('207')  SlaveDataType=uint8  DataLength=1  NoAck=off  RepeatedStart=off  OutputStatus=off
  wires:
  Constant1/1 -> Mux/2
  DATA/1 -> Mux/3
  Constant/1 -> Mux/1
  Mux/1 -> REGISTER ADDRESS/1

== system CAR_CONTROL_SYSTEM/HARDWARE/SENSORS/WALL RANGE SENSOR/VL6180X_I2C_REAR/VL6180X INITIALIZATION/LOAD PRIVATE REGISTERS (MANDATORY)/I2C WRITE: 0x1AD  ==
  DATA : Inport
  Constant : Constant  Value=REGISTER_ADDRESS_MSB  OutDataTypeStr=uint8  SampleTime=SAMPLING_TIME
  Constant1 : Constant  Value=REGISTER_ADDRESS_LSB  OutDataTypeStr=uint8  SampleTime=SAMPLING_TIME
  Mux : Mux  Inputs=3
  REGISTER ADDRESS : raspberrypiCommlib/I2C Controller Write  Priority=10  BoardProperty=Pi 3 Model B+  I2CModule=1  Mode=Master  SlaveAddress=SLAVE_ADDRESS  SlaveByteOrder=BigEndian  Direction=Transmitter  RegisterAddressMode=off  RegisterAddress=hex2dec('207')  SlaveDataType=uint8  DataLength=1  NoAck=off  RepeatedStart=off  OutputStatus=off
  wires:
  Constant1/1 -> Mux/2
  DATA/1 -> Mux/3
  Constant/1 -> Mux/1
  Mux/1 -> REGISTER ADDRESS/1

== system CAR_CONTROL_SYSTEM/HARDWARE/SENSORS/WALL RANGE SENSOR/VL6180X_I2C_REAR/VL6180X INITIALIZATION/LOAD PRIVATE REGISTERS (MANDATORY)/I2C WRITE: 0x1B0  ==
  DATA : Inport
  Constant : Constant  Value=REGISTER_ADDRESS_MSB  OutDataTypeStr=uint8  SampleTime=SAMPLING_TIME
  Constant1 : Constant  Value=REGISTER_ADDRESS_LSB  OutDataTypeStr=uint8  SampleTime=SAMPLING_TIME
  Mux : Mux  Inputs=3
  REGISTER ADDRESS : raspberrypiCommlib/I2C Controller Write  Priority=10  BoardProperty=Pi 3 Model B+  I2CModule=1  Mode=Master  SlaveAddress=SLAVE_ADDRESS  SlaveByteOrder=BigEndian  Direction=Transmitter  RegisterAddressMode=off  RegisterAddress=hex2dec('207')  SlaveDataType=uint8  DataLength=1  NoAck=off  RepeatedStart=off  OutputStatus=off
  wires:
  Constant1/1 -> Mux/2
  DATA/1 -> Mux/3
  Constant/1 -> Mux/1
  Mux/1 -> REGISTER ADDRESS/1

== system CAR_CONTROL_SYSTEM/HARDWARE/SENSORS/WALL RANGE SENSOR/VL6180X_I2C_REAR/VL6180X INITIALIZATION/LOAD PRIVATE REGISTERS (MANDATORY)/I2C WRITE: 0x207 ==
  DATA : Inport
  Constant : Constant  Value=REGISTER_ADDRESS_MSB  OutDataTypeStr=uint8  SampleTime=SAMPLING_TIME
  Constant1 : Constant  Value=REGISTER_ADDRESS_LSB  OutDataTypeStr=uint8  SampleTime=SAMPLING_TIME
  Mux : Mux  Inputs=3
  REGISTER ADDRESS : raspberrypiCommlib/I2C Controller Write  Priority=10  BoardProperty=Pi 3 Model B+  I2CModule=1  Mode=Master  SlaveAddress=SLAVE_ADDRESS  SlaveByteOrder=BigEndian  Direction=Transmitter  RegisterAddressMode=off  RegisterAddress=hex2dec('207')  SlaveDataType=uint8  DataLength=1  NoAck=off  RepeatedStart=off  OutputStatus=off
  wires:
  Constant1/1 -> Mux/2
  DATA/1 -> Mux/3
  Constant/1 -> Mux/1
  Mux/1 -> REGISTER ADDRESS/1

== system CAR_CONTROL_SYSTEM/HARDWARE/SENSORS/WALL RANGE SENSOR/VL6180X_I2C_REAR/VL6180X INITIALIZATION/LOAD PRIVATE REGISTERS (MANDATORY)/I2C WRITE: 0x208 ==
  DATA : Inport
  Constant : Constant  Value=REGISTER_ADDRESS_MSB  OutDataTypeStr=uint8  SampleTime=SAMPLING_TIME
  Constant1 : Constant  Value=REGISTER_ADDRESS_LSB  OutDataTypeStr=uint8  SampleTime=SAMPLING_TIME
  Mux : Mux  Inputs=3
  REGISTER ADDRESS : raspberrypiCommlib/I2C Controller Write  Priority=10  BoardProperty=Pi 3 Model B+  I2CModule=1  Mode=Master  SlaveAddress=SLAVE_ADDRESS  SlaveByteOrder=BigEndian  Direction=Transmitter  RegisterAddressMode=off  RegisterAddress=hex2dec('207')  SlaveDataType=uint8  DataLength=1  NoAck=off  RepeatedStart=off  OutputStatus=off
  wires:
  Constant1/1 -> Mux/2
  DATA/1 -> Mux/3
  Constant/1 -> Mux/1
  Mux/1 -> REGISTER ADDRESS/1

== system CAR_CONTROL_SYSTEM/HARDWARE/SENSORS/WALL RANGE SENSOR/VL6180X_I2C_REAR/VL6180X INITIALIZATION/LOAD PUBLIC REGISTERS (OPTIONAL)/I2C WRITE: SYSRANGE_INTERMEASUREMENT_PERIOD ==
  DATA : Inport
  Constant : Constant  Value=REGISTER_ADDRESS_MSB  OutDataTypeStr=uint8  SampleTime=SAMPLING_TIME
  Constant1 : Constant  Value=REGISTER_ADDRESS_LSB  OutDataTypeStr=uint8  SampleTime=SAMPLING_TIME
  Mux : Mux  Inputs=3
  REGISTER ADDRESS : raspberrypiCommlib/I2C Controller Write  Priority=10  BoardProperty=Pi 3 Model B+  I2CModule=1  Mode=Master  SlaveAddress=SLAVE_ADDRESS  SlaveByteOrder=BigEndian  Direction=Transmitter  RegisterAddressMode=off  RegisterAddress=hex2dec('207')  SlaveDataType=uint8  DataLength=1  NoAck=off  RepeatedStart=off  OutputStatus=off
  wires:
  Constant1/1 -> Mux/2
  DATA/1 -> Mux/3
  Constant/1 -> Mux/1
  Mux/1 -> REGISTER ADDRESS/1

== system CAR_CONTROL_SYSTEM/HARDWARE/SENSORS/WALL RANGE SENSOR/VL6180X_I2C_REAR/VL6180X INITIALIZATION/LOAD PUBLIC REGISTERS (OPTIONAL)/I2C WRITE: SYSALS_INTERMEASUREMENT_PERIOD ==
  DATA : Inport
  Constant : Constant  Value=REGISTER_ADDRESS_MSB  OutDataTypeStr=uint8  SampleTime=SAMPLING_TIME
  Constant1 : Constant  Value=REGISTER_ADDRESS_LSB  OutDataTypeStr=uint8  SampleTime=SAMPLING_TIME
  Mux : Mux  Inputs=3
  REGISTER ADDRESS : raspberrypiCommlib/I2C Controller Write  Priority=10  BoardProperty=Pi 3 Model B+  I2CModule=1  Mode=Master  SlaveAddress=SLAVE_ADDRESS  SlaveByteOrder=BigEndian  Direction=Transmitter  RegisterAddressMode=off  RegisterAddress=hex2dec('207')  SlaveDataType=uint8  DataLength=1  NoAck=off  RepeatedStart=off  OutputStatus=off
  wires:
  Constant1/1 -> Mux/2
  DATA/1 -> Mux/3
  Constant/1 -> Mux/1
  Mux/1 -> REGISTER ADDRESS/1

== system CAR_CONTROL_SYSTEM/HARDWARE/SENSORS/WALL RANGE SENSOR/VL6180X_I2C_REAR/VL6180X INITIALIZATION/LOAD PUBLIC REGISTERS (OPTIONAL)/I2C WRITE: SYSTEM_INTERRUPT_CONFIG_GPIO ==
  DATA : Inport
  Constant : Constant  Value=REGISTER_ADDRESS_MSB  OutDataTypeStr=uint8  SampleTime=SAMPLING_TIME
  Constant1 : Constant  Value=REGISTER_ADDRESS_LSB  OutDataTypeStr=uint8  SampleTime=SAMPLING_TIME
  Mux : Mux  Inputs=3
  REGISTER ADDRESS : raspberrypiCommlib/I2C Controller Write  Priority=10  BoardProperty=Pi 3 Model B+  I2CModule=1  Mode=Master  SlaveAddress=SLAVE_ADDRESS  SlaveByteOrder=BigEndian  Direction=Transmitter  RegisterAddressMode=off  RegisterAddress=hex2dec('207')  SlaveDataType=uint8  DataLength=1  NoAck=off  RepeatedStart=off  OutputStatus=off
  wires:
  Constant1/1 -> Mux/2
  DATA/1 -> Mux/3
  Constant/1 -> Mux/1
  Mux/1 -> REGISTER ADDRESS/1

== system CAR_CONTROL_SYSTEM/HARDWARE/SENSORS/WALL RANGE SENSOR/VL6180X_I2C_REAR/VL6180X INITIALIZATION/LOAD PUBLIC REGISTERS (RECOMMENDED)/I2C WRITE: READOUT_AVERAGING_SAMPLE_PERIOD ==
  DATA : Inport
  Constant : Constant  Value=REGISTER_ADDRESS_MSB  OutDataTypeStr=uint8  SampleTime=SAMPLING_TIME
  Constant1 : Constant  Value=REGISTER_ADDRESS_LSB  OutDataTypeStr=uint8  SampleTime=SAMPLING_TIME
  Mux : Mux  Inputs=3
  REGISTER ADDRESS : raspberrypiCommlib/I2C Controller Write  Priority=10  BoardProperty=Pi 3 Model B+  I2CModule=1  Mode=Master  SlaveAddress=SLAVE_ADDRESS  SlaveByteOrder=BigEndian  Direction=Transmitter  RegisterAddressMode=off  RegisterAddress=hex2dec('207')  SlaveDataType=uint8  DataLength=1  NoAck=off  RepeatedStart=off  OutputStatus=off
  wires:
  Constant1/1 -> Mux/2
  DATA/1 -> Mux/3
  Constant/1 -> Mux/1
  Mux/1 -> REGISTER ADDRESS/1

== system CAR_CONTROL_SYSTEM/HARDWARE/SENSORS/WALL RANGE SENSOR/VL6180X_I2C_REAR/VL6180X INITIALIZATION/LOAD PUBLIC REGISTERS (RECOMMENDED)/I2C WRITE: SYSALS_ANALOGUE_GAIN ==
  DATA : Inport
  Constant : Constant  Value=REGISTER_ADDRESS_MSB  OutDataTypeStr=uint8  SampleTime=SAMPLING_TIME
  Constant1 : Constant  Value=REGISTER_ADDRESS_LSB  OutDataTypeStr=uint8  SampleTime=SAMPLING_TIME
  Mux : Mux  Inputs=3
  REGISTER ADDRESS : raspberrypiCommlib/I2C Controller Write  Priority=10  BoardProperty=Pi 3 Model B+  I2CModule=1  Mode=Master  SlaveAddress=SLAVE_ADDRESS  SlaveByteOrder=BigEndian  Direction=Transmitter  RegisterAddressMode=off  RegisterAddress=hex2dec('207')  SlaveDataType=uint8  DataLength=1  NoAck=off  RepeatedStart=off  OutputStatus=off
  wires:
  Constant1/1 -> Mux/2
  DATA/1 -> Mux/3
  Constant/1 -> Mux/1
  Mux/1 -> REGISTER ADDRESS/1

== system CAR_CONTROL_SYSTEM/HARDWARE/SENSORS/WALL RANGE SENSOR/VL6180X_I2C_REAR/VL6180X INITIALIZATION/LOAD PUBLIC REGISTERS (RECOMMENDED)/I2C WRITE: SYSALS_INTEGRATION_PERIOD ==
  DATA : Inport
  Constant : Constant  Value=REGISTER_ADDRESS_MSB  OutDataTypeStr=uint8  SampleTime=SAMPLING_TIME
  Constant1 : Constant  Value=REGISTER_ADDRESS_LSB  OutDataTypeStr=uint8  SampleTime=SAMPLING_TIME
  Mux : Mux  Inputs=3
  REGISTER ADDRESS : raspberrypiCommlib/I2C Controller Write  Priority=10  BoardProperty=Pi 3 Model B+  I2CModule=1  Mode=Master  SlaveAddress=SLAVE_ADDRESS  SlaveByteOrder=BigEndian  Direction=Transmitter  RegisterAddressMode=off  RegisterAddress=hex2dec('207')  SlaveDataType=uint8  DataLength=1  NoAck=off  RepeatedStart=off  OutputStatus=off
  wires:
  Constant1/1 -> Mux/2
  DATA/1 -> Mux/3
  Constant/1 -> Mux/1
  Mux/1 -> REGISTER ADDRESS/1

== system CAR_CONTROL_SYSTEM/HARDWARE/SENSORS/WALL RANGE SENSOR/VL6180X_I2C_REAR/VL6180X INITIALIZATION/LOAD PUBLIC REGISTERS (RECOMMENDED)/I2C WRITE: SYSRANGE_VHV_RECALIBRATE ==
  DATA : Inport
  Constant : Constant  Value=REGISTER_ADDRESS_MSB  OutDataTypeStr=uint8  SampleTime=SAMPLING_TIME
  Constant1 : Constant  Value=REGISTER_ADDRESS_LSB  OutDataTypeStr=uint8  SampleTime=SAMPLING_TIME
  Mux : Mux  Inputs=3
  REGISTER ADDRESS : raspberrypiCommlib/I2C Controller Write  Priority=10  BoardProperty=Pi 3 Model B+  I2CModule=1  Mode=Master  SlaveAddress=SLAVE_ADDRESS  SlaveByteOrder=BigEndian  Direction=Transmitter  RegisterAddressMode=off  RegisterAddress=hex2dec('207')  SlaveDataType=uint8  DataLength=1  NoAck=off  RepeatedStart=off  OutputStatus=off
  wires:
  Constant1/1 -> Mux/2
  DATA/1 -> Mux/3
  Constant/1 -> Mux/1
  Mux/1 -> REGISTER ADDRESS/1

== system CAR_CONTROL_SYSTEM/HARDWARE/SENSORS/WALL RANGE SENSOR/VL6180X_I2C_REAR/VL6180X INITIALIZATION/LOAD PUBLIC REGISTERS (RECOMMENDED)/I2C WRITE: SYSRANGE_VHV_REPEAT_RATE ==
  DATA : Inport
  Constant : Constant  Value=REGISTER_ADDRESS_MSB  OutDataTypeStr=uint8  SampleTime=SAMPLING_TIME
  Constant1 : Constant  Value=REGISTER_ADDRESS_LSB  OutDataTypeStr=uint8  SampleTime=SAMPLING_TIME
  Mux : Mux  Inputs=3
  REGISTER ADDRESS : raspberrypiCommlib/I2C Controller Write  Priority=10  BoardProperty=Pi 3 Model B+  I2CModule=1  Mode=Master  SlaveAddress=SLAVE_ADDRESS  SlaveByteOrder=BigEndian  Direction=Transmitter  RegisterAddressMode=off  RegisterAddress=hex2dec('207')  SlaveDataType=uint8  DataLength=1  NoAck=off  RepeatedStart=off  OutputStatus=off
  wires:
  Constant1/1 -> Mux/2
  DATA/1 -> Mux/3
  Constant/1 -> Mux/1
  Mux/1 -> REGISTER ADDRESS/1

== system CAR_CONTROL_SYSTEM/HARDWARE/SENSORS/WALL RANGE SENSOR/VL6180X_I2C_REAR/VL6180X INITIALIZATION/LOAD PUBLIC REGISTERS (RECOMMENDED)/I2C WRITE: SYSTEM_MODE_GPIO1 ==
  DATA : Inport
  Constant : Constant  Value=REGISTER_ADDRESS_MSB  OutDataTypeStr=uint8  SampleTime=SAMPLING_TIME
  Constant1 : Constant  Value=REGISTER_ADDRESS_LSB  OutDataTypeStr=uint8  SampleTime=SAMPLING_TIME
  Mux : Mux  Inputs=3
  REGISTER ADDRESS : raspberrypiCommlib/I2C Controller Write  Priority=10  BoardProperty=Pi 3 Model B+  I2CModule=1  Mode=Master  SlaveAddress=SLAVE_ADDRESS  SlaveByteOrder=BigEndian  Direction=Transmitter  RegisterAddressMode=off  RegisterAddress=hex2dec('207')  SlaveDataType=uint8  DataLength=1  NoAck=off  RepeatedStart=off  OutputStatus=off
  wires:
  Constant1/1 -> Mux/2
  DATA/1 -> Mux/3
  Constant/1 -> Mux/1
  Mux/1 -> REGISTER ADDRESS/1

== system CAR_CONTROL_SYSTEM/HARDWARE/SENSORS/WALL RANGE SENSOR/VL6180X_I2C_REAR/VL6180X INITIALIZATION/MEASUREMENT CONFIGURATION/I2C WRITE: SYSTEM_INTERRUPT_CLEAR ==
  DATA : Inport
  Constant : Constant  Value=REGISTER_ADDRESS_MSB  OutDataTypeStr=uint8  SampleTime=SAMPLING_TIME
  Constant1 : Constant  Value=REGISTER_ADDRESS_LSB  OutDataTypeStr=uint8  SampleTime=SAMPLING_TIME
  Mux : Mux  Inputs=3
  REGISTER ADDRESS : raspberrypiCommlib/I2C Controller Write  Priority=10  BoardProperty=Pi 3 Model B+  I2CModule=1  Mode=Master  SlaveAddress=SLAVE_ADDRESS  SlaveByteOrder=BigEndian  Direction=Transmitter  RegisterAddressMode=off  RegisterAddress=hex2dec('207')  SlaveDataType=uint8  DataLength=1  NoAck=off  RepeatedStart=off  OutputStatus=off
  wires:
  Constant1/1 -> Mux/2
  DATA/1 -> Mux/3
  Constant/1 -> Mux/1
  Mux/1 -> REGISTER ADDRESS/1

== system CAR_CONTROL_SYSTEM/HARDWARE/SENSORS/WALL RANGE SENSOR/VL6180X_I2C_REAR/VL6180X INITIALIZATION/MEASUREMENT CONFIGURATION/START READ RANGE CONTINUOUS ==
  Enable : EnablePort
  Constant2 : Constant  Value=hex2dec('03')  OutDataTypeStr=uint8  SampleTime=SAMPLING_TIME
  I2C WRITE: SYSRANGE_START : Subsystem  mask{SLAVE_ADDRESS=VL6180X.ADDRESS, REGISTER_ADDRESS=VL6180X.SYSRANGE_START}
      mask prompts: SLAVE_ADDRESS "SLAVE ADDRESS"; REGISTER_ADDRESS "REGISTER ADDRESS"
      mask init:
      | REGISTER_ADDRESS_MSB = uint8(floor(REGISTER_ADDRESS/(2^8)));
      | REGISTER_ADDRESS_LSB = uint8(rem(REGISTER_ADDRESS,2^8));
  wires:
  Constant2/1 -> I2C WRITE: SYSRANGE_START/1(DATA)

== system CAR_CONTROL_SYSTEM/HARDWARE/SENSORS/WALL RANGE SENSOR/VL6180X_I2C_REAR/VL6180X INITIALIZATION/MEASUREMENT CONFIGURATION/START READ RANGE SINGLE ==
  Enable : EnablePort
  Constant1 : Constant  Value=hex2dec('01')  OutDataTypeStr=uint8  SampleTime=SAMPLING_TIME
  I2C WRITE: SYSRANGE_START : Subsystem  mask{SLAVE_ADDRESS=VL6180X.ADDRESS, REGISTER_ADDRESS=VL6180X.SYSRANGE_START}
      mask prompts: SLAVE_ADDRESS "SLAVE ADDRESS"; REGISTER_ADDRESS "REGISTER ADDRESS"
      mask init:
      | REGISTER_ADDRESS_MSB = uint8(floor(REGISTER_ADDRESS/(2^8)));
      | REGISTER_ADDRESS_LSB = uint8(rem(REGISTER_ADDRESS,2^8));
  wires:
  Constant1/1 -> I2C WRITE: SYSRANGE_START/1(DATA)

== system CAR_CONTROL_SYSTEM/HARDWARE/SENSORS/WALL RANGE SENSOR/VL6180X_I2C_REAR/VL6180X INITIALIZATION/OTHER SPECIFIC SETTINGS (OPTIONAL)/I2C WRITE: INTERLEAVED_MODE_ENABLE ==
  DATA : Inport
  Constant : Constant  Value=REGISTER_ADDRESS_MSB  OutDataTypeStr=uint8  SampleTime=SAMPLING_TIME
  Constant1 : Constant  Value=REGISTER_ADDRESS_LSB  OutDataTypeStr=uint8  SampleTime=SAMPLING_TIME
  Mux : Mux  Inputs=3
  REGISTER ADDRESS : raspberrypiCommlib/I2C Controller Write  Priority=10  BoardProperty=Pi 3 Model B+  I2CModule=1  Mode=Master  SlaveAddress=SLAVE_ADDRESS  SlaveByteOrder=BigEndian  Direction=Transmitter  RegisterAddressMode=off  RegisterAddress=hex2dec('207')  SlaveDataType=uint8  DataLength=1  NoAck=off  RepeatedStart=off  OutputStatus=off
  wires:
  Constant1/1 -> Mux/2
  DATA/1 -> Mux/3
  Constant/1 -> Mux/1
  Mux/1 -> REGISTER ADDRESS/1

== system CAR_CONTROL_SYSTEM/HARDWARE/SENSORS/WALL RANGE SENSOR/VL6180X_I2C_REAR/VL6180X INITIALIZATION/OTHER SPECIFIC SETTINGS (OPTIONAL)/I2C WRITE: SYSRANGE_MAX_CONVERGENCE_TIME ==
  DATA : Inport
  Constant : Constant  Value=REGISTER_ADDRESS_MSB  OutDataTypeStr=uint8  SampleTime=SAMPLING_TIME
  Constant1 : Constant  Value=REGISTER_ADDRESS_LSB  OutDataTypeStr=uint8  SampleTime=SAMPLING_TIME
  Mux : Mux  Inputs=3
  REGISTER ADDRESS : raspberrypiCommlib/I2C Controller Write  Priority=10  BoardProperty=Pi 3 Model B+  I2CModule=1  Mode=Master  SlaveAddress=SLAVE_ADDRESS  SlaveByteOrder=BigEndian  Direction=Transmitter  RegisterAddressMode=off  RegisterAddress=hex2dec('207')  SlaveDataType=uint8  DataLength=1  NoAck=off  RepeatedStart=off  OutputStatus=off
  wires:
  Constant1/1 -> Mux/2
  DATA/1 -> Mux/3
  Constant/1 -> Mux/1
  Mux/1 -> REGISTER ADDRESS/1

== system CAR_CONTROL_SYSTEM/HARDWARE/SENSORS/WALL RANGE SENSOR/VL6180X_I2C_FRONT/VL6180X INITIALIZATION/MEASUREMENT CONFIGURATION/START READ RANGE CONTINUOUS/I2C WRITE: SYSRANGE_START ==
  DATA : Inport
  Constant : Constant  Value=REGISTER_ADDRESS_MSB  OutDataTypeStr=uint8  SampleTime=SAMPLING_TIME
  Constant1 : Constant  Value=REGISTER_ADDRESS_LSB  OutDataTypeStr=uint8  SampleTime=SAMPLING_TIME
  Mux : Mux  Inputs=3
  REGISTER ADDRESS : raspberrypiCommlib/I2C Controller Write  Priority=10  BoardProperty=Pi 3 Model B+  I2CModule=1  Mode=Master  SlaveAddress=SLAVE_ADDRESS  SlaveByteOrder=BigEndian  Direction=Transmitter  RegisterAddressMode=off  RegisterAddress=hex2dec('207')  SlaveDataType=uint8  DataLength=1  NoAck=off  RepeatedStart=off  OutputStatus=off
  wires:
  Mux/1 -> REGISTER ADDRESS/1
  Constant/1 -> Mux/1
  DATA/1 -> Mux/3
  Constant1/1 -> Mux/2
